simulink model "controllo_motore"  (R2024b)
settings: Solver=ode15s  StartTime=0.0  StopTime=5.3333  MaxStep=1e-3  RelTol=1e-3
undefined symbols (not defined in the file): AmpiezzaRumorePercentuale, anti_wind_up, Beta, coppia_carico, DeadZoneCorrente, Gnd, High_voltage, input_ramp_slope, input_step_amplitude, J_macchina, J_motore, k_deamp, kamp, kdt, kff, ki, kp, kt, kv, La, Nlamelle, noise_on, R_rid, Ra, saturazione_contr_high, saturazione_contr_low, Va, w_max_rad_s
libraries: simulink x1
settings Model: Creator=USER  LastModifiedBy=USER
settings SolverCC: AlgebraicLoopSolver=TrustRegion
settings DebuggingCC: InheritedTsInSrcMsg=none  UnconnectedInputMsg=warning  UnconnectedOutputMsg=warning  UnconnectedLineMsg=warning
settings ModelReferenceCC: EnableRefExpFcnMdlSchedulingChecks=on
settings RTWCC: GPUComputeCapability=3.5  DLArmComputeVersion=19.05

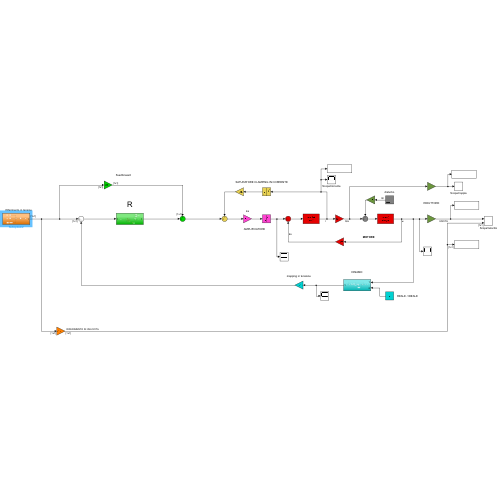
[thumbnail: Simulink's stored preview of the top-level diagram]
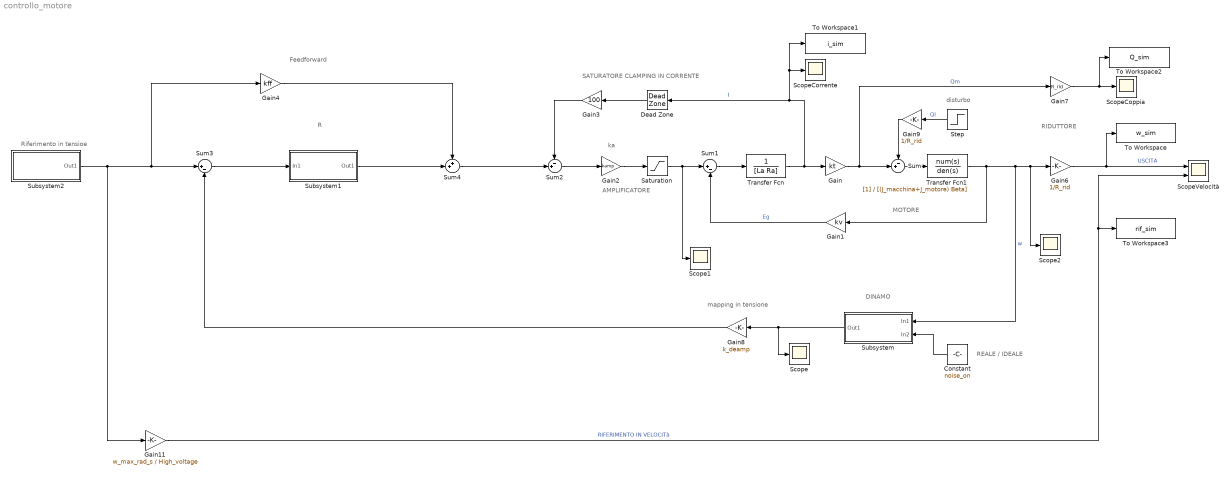
== system controllo_motore ==
  note: disturbo
  note: Feedforward
  note: Riferimento in tensioe
  note: R
  note: mapping in tensione
  note: REALE / IDEALE
  note: ka
  note: MOTORE
  note: SATURATORE CLAMPING IN CORRENTE
  note: AMPLIFICATORE
  note: DINAMO
  note: RIDUTTORE
  Constant : Constant  Value=noise_on
  Dead Zone : DeadZone  LowerValue=-DeadZoneCorrente  UpperValue=DeadZoneCorrente
  Gain : Gain  Gain=kt
  Gain1 : Gain  Gain=kv
  Gain11 : Gain  Gain=w_max_rad_s / High_voltage
  Gain2 : Gain  Gain=kamp
  Gain3 : Gain  Gain=100
  Gain4 : Gain  Gain=kff
  Gain6 : Gain  Gain=1/R_rid
  Gain7 : Gain  Gain=R_rid
  Gain8 : Gain  Gain=k_deamp
  Gain9 : Gain  Gain=1/R_rid
  Saturation : Saturate  UpperLimit=Va  LowerLimit=Gnd
  Scope : Scope
  Scope1 : Scope
  Scope2 : Scope
  ScopeCoppia : Scope
  ScopeCorrente : Scope
  ScopeVelocità : Scope  NumInputPorts=2
  Step : Step  After=coppia_carico  SampleTime=0
  Subsystem : Subsystem
  Subsystem1 : Subsystem
  Subsystem2 : Subsystem
  Sum : Sum  Inputs=-+|
  Sum1 : Sum  Inputs=|+-
  Sum2 : Sum  Inputs=-+|
  Sum3 : Sum  Inputs=|+-
  Sum4 : Sum  Inputs=++|
  To Workspace : ToWorkspace  VariableName=w_sim  SaveFormat=Timeseries  SampleTime=-1
  To Workspace1 : ToWorkspace  VariableName=i_sim  SaveFormat=Timeseries  SampleTime=-1
  To Workspace2 : ToWorkspace  VariableName=Q_sim  SaveFormat=Timeseries  SampleTime=-1
  To Workspace3 : ToWorkspace  VariableName=rif_sim  SaveFormat=Timeseries  SampleTime=-1
  Transfer Fcn : TransferFcn  Denominator=[La Ra]
  Transfer Fcn1 : TransferFcn  Denominator=[(J_macchina+J_motore) Beta]
  wires:
  Sum1/1 -> Transfer Fcn/1
  Gain1/1 -> Sum1/2  "Eg"
  Gain/1 -> Gain7/1, Sum/2  "Qm"
  Transfer Fcn1/1 -> Subsystem/1(In1), Scope2/1, Gain6/1, Gain1/1  "w"
  Sum/1 -> Transfer Fcn1/1
  Transfer Fcn/1 -> To Workspace1/1, ScopeCorrente/1, Dead Zone/1, Gain/1  "I"
  Gain2/1 -> Saturation/1
  Saturation/1 -> Scope1/1, Sum1/1
  Dead Zone/1 -> Gain3/1
  Gain3/1 -> Sum2/1
  Sum2/1 -> Gain2/1
  Gain6/1 -> To Workspace/1, ScopeVelocità/1  "USCITA"
  Gain7/1 -> To Workspace2/1, ScopeCoppia/1
  Subsystem/1(Out1) -> Scope/1, Gain8/1
  Gain8/1 -> Sum3/2
  Subsystem2/1(Out1) -> Sum3/1, Gain4/1, Gain11/1
  Step/1 -> Gain9/1  "Ql"
  Gain9/1 -> Sum/1
  Gain11/1 -> To Workspace3/1, ScopeVelocità/2  "RIFERIMENTO IN VELOCITà"
  Constant/1 -> Subsystem/2(In2)
  Sum3/1 -> Subsystem1/1(In1)
  Subsystem1/1(Out1) -> Sum4/2
  Gain4/1 -> Sum4/1
  Sum4/1 -> Sum2/2

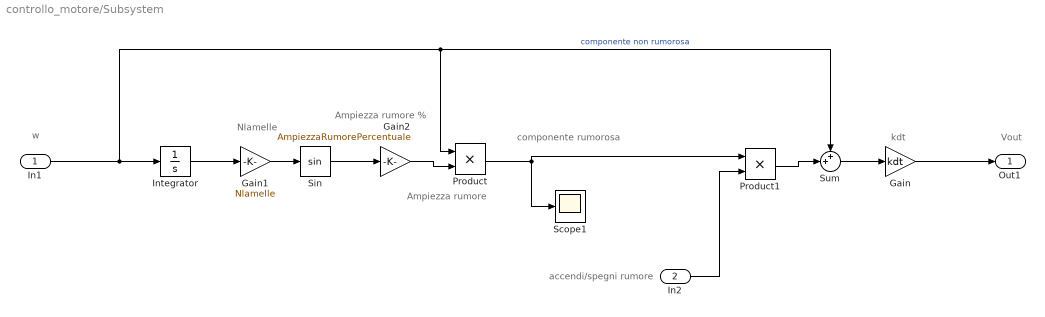
== system controllo_motore/Subsystem ==
  note: componente rumorosa
  note: Ampiezza rumore
  note: w
  note: Vout
  note: kdt
  note: Nlamelle
  note: Ampiezza rumore %
  note: accendi/spegni rumore
  In1 : Inport
  In2 : Inport  Port=2
  Gain : Gain  Gain=kdt
  Gain1 : Gain  Gain=Nlamelle
  Gain2 : Gain  Gain=AmpiezzaRumorePercentuale
  Integrator : Integrator
  Product : Product
  Product1 : Product
  Scope1 : Scope
  Sin : Trigonometry
  Sum : Sum  Inputs=++|
  Out1 : Outport
  wires:
  Sum/1 -> Gain/1
  Gain/1 -> Out1/1
  Gain1/1 -> Sin/1
  Integrator/1 -> Gain1/1
  Sin/1 -> Gain2/1
  In1/1 -> Product/1, Sum/1, Integrator/1  "componente non rumorosa"
  Gain2/1 -> Product/2
  Product/1 -> Product1/1, Scope1/1
  Product1/1 -> Sum/2
  In2/1 -> Product1/2

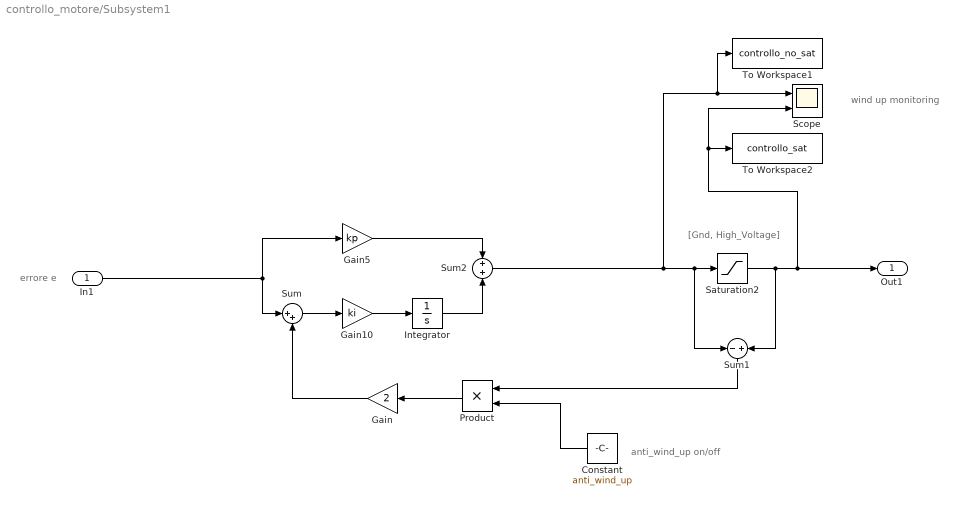
== system controllo_motore/Subsystem1 ==
  note: [Gnd, High_Voltage]
  note: wind up monitoring
  note: anti_wind_up on/off
  note: errore e
  In1 : Inport
  Constant : Constant  Value=anti_wind_up
  Gain : Gain  Gain=2
  Gain10 : Gain  Gain=ki
  Gain5 : Gain  Gain=kp
  Integrator : Integrator
  Product : Product
  Saturation2 : Saturate  UpperLimit=saturazione_contr_high  LowerLimit=saturazione_contr_low
  Scope : Scope  NumInputPorts=2
  Sum : Sum  Inputs=|++
  Sum1 : Sum  Inputs=-|+
  Sum2 : Sum  Inputs=+|+
  To Workspace1 : ToWorkspace  VariableName=controllo_no_sat  SaveFormat=Timeseries  SampleTime=-1
  To Workspace2 : ToWorkspace  VariableName=controllo_sat  SaveFormat=Timeseries  SampleTime=-1
  Out1 : Outport
  wires:
  In1/1 -> Gain5/1, Sum/1
  Gain10/1 -> Integrator/1
  Sum2/1 -> Saturation2/1, Sum1/1, To Workspace1/1, Scope/1
  Saturation2/1 -> To Workspace2/1, Scope/2, Out1/1, Sum1/2
  Sum/1 -> Gain10/1
  Sum1/1 -> Product/1
  Constant/1 -> Product/2
  Product/1 -> Gain/1
  Gain/1 -> Sum/2
  Integrator/1 -> Sum2/2
  Gain5/1 -> Sum2/1

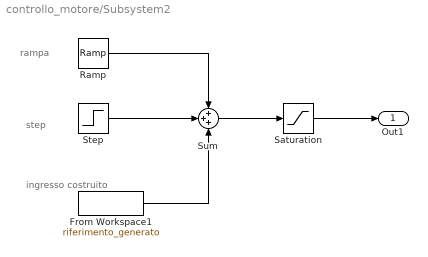
== system controllo_motore/Subsystem2 ==
  note: ingresso
      | costruito
  note: step
  note: rampa
  From Workspace1 : FromWorkspace  VariableName=riferimento_generato  SampleTime=-1
  Ramp : simulink/Sources/Ramp  slope=input_ramp_slope  start=1  InitialOutput=0
  Saturation : Saturate  UpperLimit=High_voltage  LowerLimit=Gnd
  Step : Step  After=input_step_amplitude  SampleTime=0
  Sum : Sum  Inputs=+++
  Out1 : Outport
  wires:
  Ramp/1 -> Sum/1
  Step/1 -> Sum/2
  Sum/1 -> Saturation/1
  Saturation/1 -> Out1/1
  From Workspace1/1 -> Sum/3
